simulink model "modele"  (R2023b)
settings: Solver=VariableStepAuto  StartTime=0.0  StopTime=10.0  MaxStep=0.01  RelTol=1e-3
undefined symbols (not defined in the file): delta_fmw, fmw_0, t_fmw, T_wew0
libraries: cstblocks x2
settings Model: Creator=tomasz  LastModifiedBy=tomasz

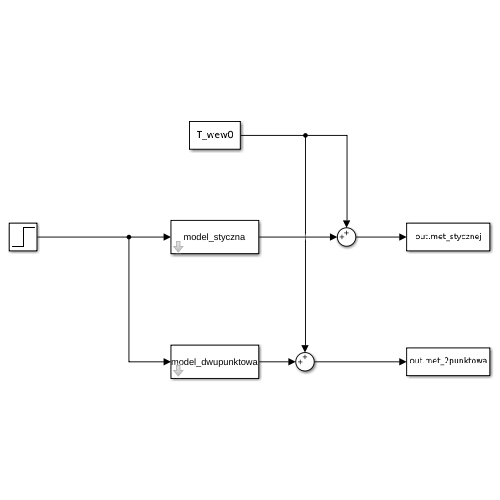
[thumbnail: Simulink's stored preview of the top-level diagram]
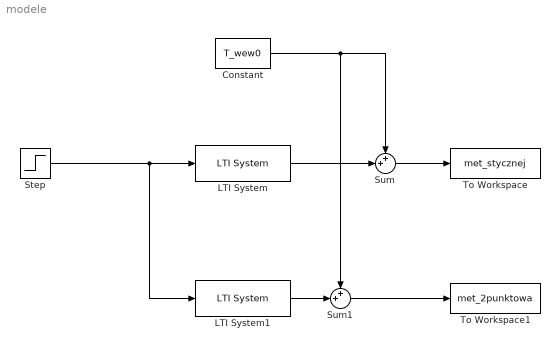
== system modele ==
  Constant : Constant  Value=T_wew0
  LTI System : cstblocks/LTI System  sys=model_styczna  IC=[]  PadeOrder=0
  LTI System1 : cstblocks/LTI System  sys=model_dwupunktowa  IC=[]  PadeOrder=0
  Step : Step  Time=t_fmw  Before=fmw_0  After=fmw_0 + delta_fmw  SampleTime=0
  Sum : Sum  Inputs=++|
  Sum1 : Sum  Inputs=++|
  To Workspace : ToWorkspace  VariableName=met_stycznej  SampleTime=-1
      settings: Save2DSignal=2-D array (concatenate along first dimension)
  To Workspace1 : ToWorkspace  VariableName=met_2punktowa  SampleTime=-1
      settings: Save2DSignal=2-D array (concatenate along first dimension)
  wires:
  LTI System/1 -> Sum/2
  Constant/1 -> Sum1/1, Sum/1
  LTI System1/1 -> Sum1/2
  Step/1 -> LTI System1/1, LTI System/1
  Sum/1 -> To Workspace/1
  Sum1/1 -> To Workspace1/1
